simulink model "Main"  (R2020b)
settings: Solver=FixedStepAuto  StartTime=0.0  StopTime=1  FixedStep=0.01  RelTol=1e-3
settings Model: Creator=kaebi  LastModifiedBy=kaebi

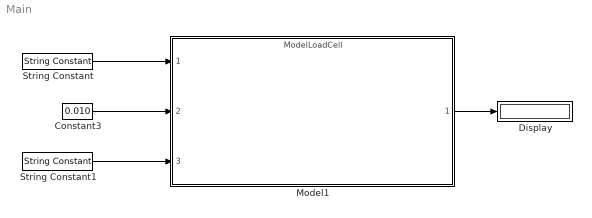
== system Main ==
  Constant3 : Constant  Value=0.010
  Display : Display
  Model1 : ModelReference  ModelNameDialog=ModelLoadCell.slx  SimulationMode=Normal  ModelReferenceVersion=1.27
  String Constant : StringConstant  String="\"Cell \""
  String Constant1 : StringConstant  String="\" g\""
  wires:
  Model1/1 -> Display/1
  Constant3/1 -> Model1/2
  String Constant/1 -> Model1/1
  String Constant1/1 -> Model1/3
